simulink model "ZVD_sythesis"  (R2018b)
settings: Solver=VariableStepAuto  StartTime=0.0  StopTime=0.05  MaxStep=1e-6  RelTol=1e-8
settings Model: Creator=secklesa  LastModifiedBy=secklesa

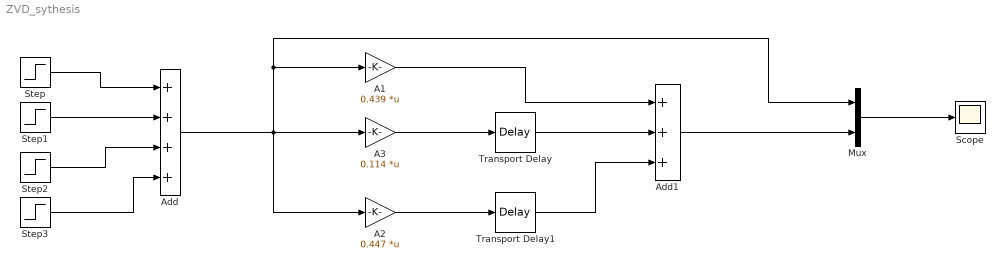
== system ZVD_sythesis ==
  A1 : Gain  Gain=0.439  Multiplication=Matrix(K*u)
  A2 : Gain  Gain=0.447  Multiplication=Matrix(K*u)
  A3 : Gain  Gain=0.114  Multiplication=Matrix(K*u)
  Add : Sum  Inputs=++++
  Add1 : Sum  Inputs=+++
  Mux : Mux  Inputs=2
  Scope : Scope
  Step : Step  Time=5E-3  SampleTime=0
  Step1 : Step  Time=15E-3  SampleTime=0
  Step2 : Step  Time=25E-3  After=-1  SampleTime=0
  Step3 : Step  Time=35E-3  After=-1  SampleTime=0
  Transport Delay : TransportDelay  DelayTime=0.001
  Transport Delay1 : TransportDelay  DelayTime=0.002
  wires:
  Step1/1 -> Add/2
  Step/1 -> Add/1
  Step2/1 -> Add/3
  Step3/1 -> Add/4
  Add/1 -> Mux/1, A1/1, A2/1, A3/1
  A3/1 -> Transport Delay/1
  A2/1 -> Transport Delay1/1
  Transport Delay1/1 -> Add1/3
  Transport Delay/1 -> Add1/2
  A1/1 -> Add1/1
  Add1/1 -> Mux/2
  Mux/1 -> Scope/1
